simulink model "Matlab2SimulinkUDPSim"  (R2020b)
settings: Solver=VariableStepAuto  StartTime=0.0  StopTime=100000  RelTol=1e-3
libraries: dspnetwork x4, sldrtlib x1
settings Model: Creator=ayurkewi  LastModifiedBy=Wacom hrg
settings DataIOCC: ReturnWorkspaceOutputs=off
settings DebuggingCC: ArithmeticOperatorsInVariantConditions=warning
settings SFSimCC: CustomCodeUndefinedFunction=UseInterfaceOnly

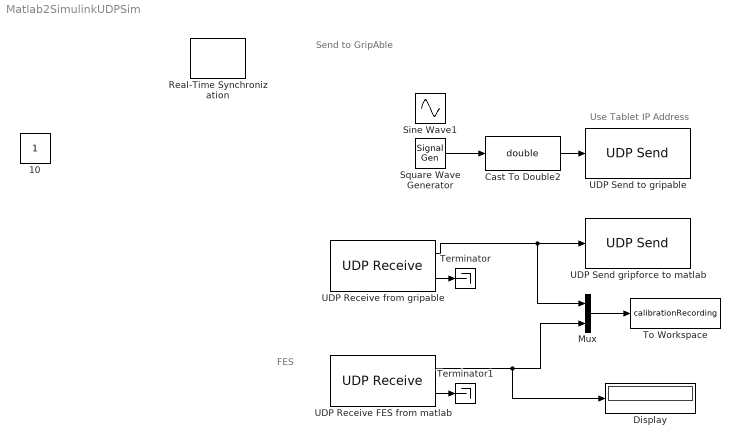
== system Matlab2SimulinkUDPSim ==
  note: Send to GripAble
  note: FES
  note: Use Tablet IP Address
  Cast To Double2 : DataTypeConversion  OutDataTypeStr=double
  Display : Display
  Mux : Mux  Inputs=2
  Real-Time Synchronization : sldrtlib/Real-Time Synchronization  SampleTime=0.001  MaxMissedTicks=100000  ShowMissedTicks=off  YieldWhenWaiting=off
  Sine Wave1 : Sin  Amplitude=2  Bias=-.2  Frequency=0.01  SampleTime=0
  Square Wave Generator : SignalGenerator  WaveForm=square  Amplitude=2  Frequency=0.1  Units=rad/sec
  Terminator : Terminator
  Terminator1 : Terminator
  To Workspace : ToWorkspace  VariableName=calibrationRecording  SaveFormat=Timeseries  SampleTime=-1
  UDP Receive FES from matlab : dspnetwork/UDP Receive  localURL='0.0.0.0'  localPort=5000  remoteURL='0.0.0.0'  remotePort=-1  recvBufferSize=8192  dims=1  signalDatatype=double  isComplex=off  isVarSize=off  showBlockingTime=off  blockingTime=0  sampletime=0.001  blockPlatform=[]
  UDP Receive from gripable : dspnetwork/UDP Receive  localURL='0.0.0.0'  localPort=26000  remoteURL='0.0.0.0'  remotePort=-1  recvBufferSize=8192  dims=1  signalDatatype=double  isComplex=off  isVarSize=off  showBlockingTime=off  blockingTime=0  sampletime=0.001  blockPlatform=[]
  UDP Send gripforce to matlab : dspnetwork/UDP Send  remoteURL='127.0.0.1'  remotePort=15000  localURL='0.0.0.0'  localPortSource=Automatically determine  localPort=-1  sendBufferSize=8192  sampletime=-1  blockPlatform=[]  separateLengthPort=0
  UDP Send to gripable : dspnetwork/UDP Send  remoteURL='146.169.201.205'  remotePort=25000  localURL='0.0.0.0'  localPortSource=Automatically determine  localPort=-1  sendBufferSize=8192  sampletime=-1  blockPlatform=[]  separateLengthPort=0
  10 : Constant  IOType=siggen
  wires:
  UDP Receive FES from matlab/1 -> Display/1, Mux/2
  UDP Receive FES from matlab/2 -> Terminator1/1
  Cast To Double2/1 -> UDP Send to gripable/1
  Square Wave Generator/1 -> Cast To Double2/1
  Mux/1 -> To Workspace/1
  UDP Receive from gripable/1 -> Mux/1, UDP Send gripforce to matlab/1
  UDP Receive from gripable/2 -> Terminator/1
